simulink model "Md61StEnCtrl"  (R2018b)
settings: Solver=FixedStepDiscrete  StartTime=0.0  StopTime=10.0  RelTol=1e-3
undefined symbols (not defined in the file or in its folder): data, KeSMSuFirstRwStBackPosDelta_Val, KeSMSuThrdRwCushFoldPosDelta_Val, KeSMSwAcsMd30PassStFldUpwdDnwdPos1_Val, KeSMSwAcsMd30PassStFrwdBkwdPos1_Val, KeSMSwAcsMd31PassStBkReclnUpwdDnwdPos1_Val, KeSMSwSeatBkLimitPos_Val, KeSMSwSeatBkLimitPosDelt_Val, PassStBkReclnEn_Clear, PassStBkReclnEn_Set, PassStCshnFldEn_Clear, PassStCshnFldEn_Set, PassStFwdBkwdEn_Clear, PassStFwdBkwdEn_Set, SecRwLtStBkReclnEn_Clear, SecRwLtStBkReclnEn_Set, SecRwLtStFwdBkwdEn_Clear, SecRwLtStFwdBkwdEn_Set, SecRwLtStLgrstInwdOtwdEn_Clear, SecRwLtStLgrstInwdOtwdEn_Set, SecRwLtStLgrstUpwdDnwdEn_Clear, SecRwLtStLgrstUpwdDnwdEn_Set, SecRwRtStBkReclnEn_Clear, SecRwRtStBkReclnEn_Set, SecRwRtStFwdBkwdEn_Clear, SecRwRtStFwdBkwdEn_Set, SecRwRtStLgrstInwdOtwdEn_Clear, SecRwRtStLgrstInwdOtwdEn_Set, SecRwRtStLgrstUpwdDnwdEn_Clear, SecRwRtStLgrstUpwdDnwdEn_Set, ThdRwLtStBkReclnEn_Clear, ThdRwLtStBkReclnEn_Set, ThdRwLtStCshnFldEn_Clear, ThdRwLtStCshnFldEn_Set, ThdRwLtStFwdBkwdEn_Clear, ThdRwLtStFwdBkwdEn_Set, ThdRwRtStBkReclnEn_Clear, ThdRwRtStBkReclnEn_Set, ThdRwRtStCshnFldEn_Clear, ThdRwRtStCshnFldEn_Set, ThdRwRtStFwdBkwdEn_Clear, ThdRwRtStFwdBkwdEn_Set, ZeroLEn_Clear, ZeroLEn_Set, ZeroREn_Clear, ZeroREn_Set
libraries: simulink x1
(part 2 of 3)

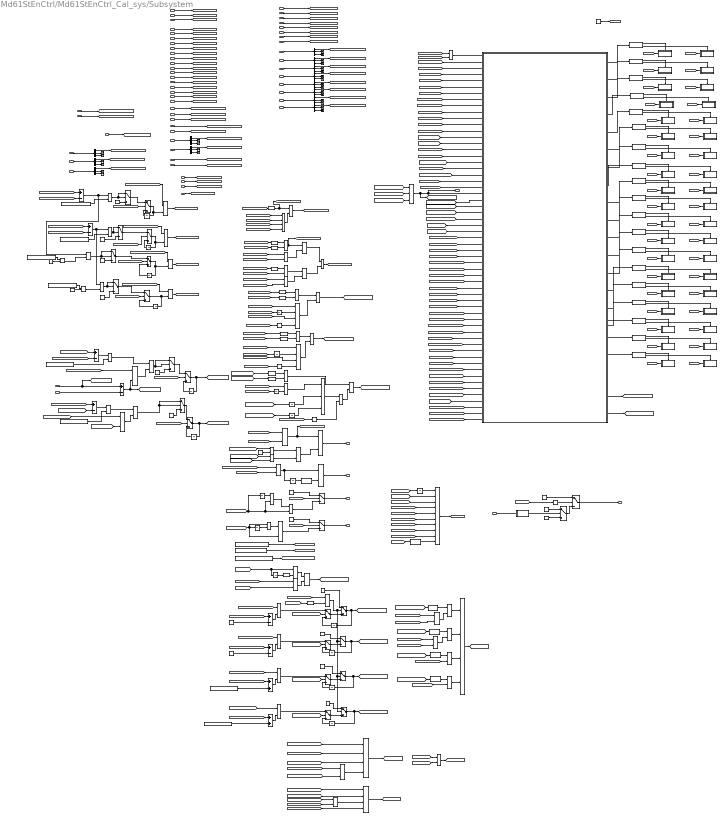
== system Md61StEnCtrl/Md61StEnCtrl_Cal_sys/Subsystem ==
  note: 3.13.1
  note: 3.13.1新增条件
  note: 3.13.1
  MdXXIsTargetPosZone_Val_read : Inport
  PassStBkReclnStgDone_Val_read : Inport  Port=2
  PassStCshnFldStgDone_Val_read : Inport  Port=3
  PassStFwdBkwdStgDone_Val_read : Inport  Port=4
  SecRwLtStBkReclnStgDone_Val_read : Inport  Port=5
  SecRwLtStFrwdBkwdStgDone_Val_read : Inport  Port=6
  SecRwLtStLgrstOtwdInwdStgDone_Val_read : Inport  Port=7
  SecRwLtStLgrstUpwdDnwdStgDone_Val_read : Inport  Port=8
  SecRwRtStBkReclnStgDone_Val_read : Inport  Port=9
  SecRwRtStFrwdBkwdStgDone_Val_read : Inport  Port=10
  SecRwRtStLgrstOtwdInwdStgDone_Val_read : Inport  Port=11
  SecRwRtStLgrstUpwdDnwdStgDone_Val_read : Inport  Port=12
  ThdRwLtStBkReclnStgDone_Val_read : Inport  Port=13
  ThdRwLtStCshnFldStgDone_Val_read : Inport  Port=14
  ThdRwLtStFwdBkwdStgDone_Val_read : Inport  Port=15
  ThdRwRtStBkReclnStgDone_Val_read : Inport  Port=16
  ThdRwRtStCshnFldStgDone_Val_read : Inport  Port=17
  ThdRwRtStFwdBkwdStgDone_Val_read : Inport  Port=18
  ZeroLStgDone_Val_read : Inport  Port=19
  ZeroRStgDone_Val_read : Inport  Port=20
  IfVeSMSbThdRwLtStCshnFldUpwdDnwdMovConfig_Val_read : Inport  Port=21
  IfVeSMSbThdRwRtStCshnFldUpwdDnwdMovConfig_Val_read : Inport  Port=22
  IfVeSMSuPassStFldUpwdDnwdPos_Val_read : Inport  Port=23
  IfVeSMSuPassStFrwdBkwdPos_Val_read : Inport  Port=24
  IfVeSMSuThdRwLtStCshnFldUpwdDnwdPos_Val_read : Inport  Port=25
  IfVeSMSuThdRwLtStFrwdBkwdPos_Val_read : Inport  Port=26
  IfVeSMSuThdRwRtStCshnFldUpwdDnwdPos_Val_read : Inport  Port=27
  IfVeSMSuThdRwRtStFrwdBkwdPos_Val_read : Inport  Port=28
  Md61ThdRwLtStCshnFldTrgtPosCalib_TrgtPosArray_read : Inport  Port=29
  Md61ThdRwRtStCshnFldTrgtPosCalib_TrgtPosArray_read : Inport  Port=30
  Md61PassStNeedFldOpn_Val_read : Inport  Port=31
  Md61ThdRwLtStNeedFldOpn_Val_read : Inport  Port=32
  Md61ThdRwRtStNeedFldOpn_Val_read : Inport  Port=33
  FirstTrig : Inport  Port=34
  KeSMSwSeatBkLimitPos_Val : Inport  Port=35
  KeSMSwSeatBkLimitPosDelt_Val : Inport  Port=36
  IfVeSMSuPassStBkReclnUpwdDnwdPos_Val_read : Inport  Port=37
  Md61PassStBkReclnTrgtPos_Val_read : Inport  Port=38
  Md61PassStFwdBkwdTrgtPosCalib_TrgtPosArray_read : Inport  Port=39
  Md61ThdRwLtStFrwdBkwdPosTrgtPosCalib_TrgtPosArray_read : Inport  Port=40
  Md61ThdRwRtStFrwdBkwdPosTrgtPosCalib_TrgtPosArray_read : Inport  Port=41
  IfVeSMSuSecRwLtStBkReclnUpwdDnwdPos_Val_read : Inport  Port=42
  IfVeSMSuSecRwLtStLgrstOtwdInwdPos_Val_read : Inport  Port=43
  IfVeSMSuSecRwLtStLgrstUpwdDnwdPos_Val_read : Inport  Port=44
  IfVeSMSuSecRwLtStZeroPos_Val_read : Inport  Port=45
  IfVeSMSuSecRwRtStBkReclnUpwdDnwdPos_Val_read : Inport  Port=46
  IfVeSMSuSecRwRtStLgrstOtwdInwdPos_Val_read : Inport  Port=47
  IfVeSMSuSecRwRtStLgrstUpwdDnwdPos_Val_read : Inport  Port=48
  IfVeSMSuSecRwRtStZeroPos_Val_read : Inport  Port=49
  Md61SecRwLtStBkReclnTrgtPosCalib_TrgtPosArray_read : Inport  Port=50
  Md61SecRwLtStCushFrntTrgtPosCalib_TrgtPosArray_read : Inport  Port=51
  Md61SecRwLtStLgrstInwdOtwdTrgtPosCalib_TrgtPosArray_read : Inport  Port=52
  Md61SecRwLtStLgrstUpwdDnwdTrgtPosCalib_TrgtPosArray_read : Inport  Port=53
  Md61SecRwRtStBkReclnTrgtPosCalib_TrgtPosArray_read : Inport  Port=54
  Md61SecRwRtStCushFrntTrgtPosCalib_TrgtPosArray_read : Inport  Port=55
  Md61SecRwRtStLgrstInwdOtwdTrgtPosCalib_TrgtPosArray_read : Inport  Port=56
  Md61SecRwRtStLgrstUpwdDnwdTrgtPosCalib_TrgtPosArray_read : Inport  Port=57
  32BitSelector1 : Subsystem  mask(32 Bit Selector){BitNum=5}
      mask prompts: BitNum "Select Bit Number"
      mask help: Allows selection of a particular bit (0-31) out of a packed word up to 32 bits long. Output will be true if the bit number selected via the mask parameter is equal to one.
      mask TypeOptions BitNum: 0 | 1 | 2 | 3 | 4 | 5 | 6 | 7 | 8 | 9 | 10 | 11 | 12 | 13 | 14 | 15 | 16 | 17 | 18 | 19 | 20 | 21 | 22 | 23 | 24 | 25 | 26 | 27 | 28 | 29 | 30 | 31
      mask Display:
      | text(0.5, 0.8,'BIT','horizontalAlignment','center')
      | text(0.5, 0.5,'SELECTOR','horizontalAlignment','center')
      | text(0.5, 0.2,['-- Bit ',char(get_param(gcb,'BitNum')),' --'],'horizontalAlignment','center')
  Add{,1,3..5,7} (6 alike) : Sum  Inputs=+-  AccumDataTypeStr=int16  OutDataTypeStr=int16
  Add2 : Sum  Inputs=+-  OutDataTypeStr=int16
  Add6 : Sum  OutDataTypeStr=int16
  Add8 : Sum  OutDataTypeStr=int16
  Chart : Stateflow chart  TreatAsAtomicUnit=on
  Constant : Constant  OutDataTypeStr=uint8
  Constant1 : Constant  Value=2  OutDataTypeStr=uint8
  Constant{10..11,16..20,22..26} (12 alike) : Constant  Value=0  OutDataTypeStr=boolean
  Constant12 : Constant  Value=120  OutDataTypeStr=int16
  Constant13 : Constant  Value=120  OutDataTypeStr=int16
  Constant2 : Constant  Value=0  OutDataTypeStr=uint8
  Constant3 : Constant  Value=5  OutDataTypeStr=uint8
  Constant4 : Constant  Value=-1  OutDataTypeStr=int16
  Constant5 : Constant  Value=-1  OutDataTypeStr=int16
  Constant9 : Constant  Value=120  OutDataTypeStr=uint16
  Demux{,1..12} (13 alike) : Demux  Outputs=3
  Divide : Product  Inputs=**  OutDataTypeStr=int16
  Divide1 : Product  Inputs=**  OutDataTypeStr=int16
  If{1..19} (19 alike) : If  IfExpression=u1
  Logical Operator{,6,11,21,26,41,51..54,68,74} (12 alike) : Logic  Operator=OR  AllPortsSameDT=off  OutDataTypeStr=boolean
  Logical Operator{1,3..4,7,10,22..23,27..28,34..35,42,46..47,49..50,55..57,70..72} (22 alike) : Logic  Operator=NOT  AllPortsSameDT=off  OutDataTypeStr=boolean
  Logical Operator{5,8..9,12..19,24,31..33,37,39..40,43..45,48,58..59,62,64..65,67,69,73} (30 alike) : Logic  AllPortsSameDT=off  OutDataTypeStr=boolean
  Logical Operator{2,20,25,60..61,63} (6 alike) : Logic  Inputs=4  AllPortsSameDT=off  OutDataTypeStr=boolean
  Logical Operator36 : Logic  Operator=OR  Inputs=3  AllPortsSameDT=off  OutDataTypeStr=boolean
  Logical Operator38 : Logic  Inputs=3  AllPortsSameDT=off  OutDataTypeStr=boolean
  Logical Operator66 : Logic  Inputs=10  AllPortsSameDT=off  OutDataTypeStr=boolean
  PA_KeSMSuFirstRwStBackPosDelta_Val{,1..3} (4 alike) : Constant  Value=KeSMSuFirstRwStBackPosDelta_Val
  PA_KeSMSuThrdRwCushFoldPosDelta_Val{,1..3} (4 alike) : Constant  Value=KeSMSuThrdRwCushFoldPosDelta_Val
  PA_KeSMSwAcsMd30PassStFldUpwdDnwdPos1_Val : Constant  Value=KeSMSwAcsMd30PassStFldUpwdDnwdPos1_Val
  PA_KeSMSwAcsMd30PassStFrwdBkwdPos1_Val : Constant  Value=KeSMSwAcsMd30PassStFrwdBkwdPos1_Val
  PA_KeSMSwAcsMd31PassStBkReclnUpwdDnwdPos1_Val : Constant  Value=KeSMSwAcsMd31PassStBkReclnUpwdDnwdPos1_Val
  PassStBkRecln_Clear : Subsystem  TreatAsAtomicUnit=on
  PassStBkRecln_Set : Subsystem  TreatAsAtomicUnit=on
  PassStCshnFld_Clear : Subsystem  TreatAsAtomicUnit=on
  PassStCshnFld_Set : Subsystem  TreatAsAtomicUnit=on
  PassStFwdBkwd_Clear : Subsystem  TreatAsAtomicUnit=on
  PassStFwdBkwd_Set : Subsystem  TreatAsAtomicUnit=on
  Relational Operator{,1,4,14..16} (6 alike) : RelationalOperator  Operator=>  OutDataTypeStr=boolean  RndMeth=Simplest
  Relational Operator10 : RelationalOperator  Operator=~=  OutDataTypeStr=boolean  RndMeth=Simplest
  Relational Operator11 : RelationalOperator  Operator=~=  OutDataTypeStr=boolean  RndMeth=Simplest
  Relational Operator{2..3,5..6,12..13} (6 alike) : RelationalOperator  Operator=<  OutDataTypeStr=boolean  RndMeth=Simplest
  Relational Operator7 : RelationalOperator  Operator=<=  OutDataTypeStr=boolean  RndMeth=Simplest
  Relational Operator8 : RelationalOperator  OutDataTypeStr=boolean  RndMeth=Simplest
  Relational Operator9 : RelationalOperator  Operator=<=  OutDataTypeStr=boolean  RndMeth=Simplest
  SecRwLtStBkRecln_Clear : Subsystem  TreatAsAtomicUnit=on
  SecRwLtStBkRecln_Set : Subsystem  TreatAsAtomicUnit=on
  SecRwLtStFwdBkwd_Clear : Subsystem  TreatAsAtomicUnit=on
  SecRwLtStFwdBkwd_Set : Subsystem  TreatAsAtomicUnit=on
  SecRwLtStLgrstInwdOtwd_Clear : Subsystem  TreatAsAtomicUnit=on
  SecRwLtStLgrstInwdOtwd_Set : Subsystem  TreatAsAtomicUnit=on
  SecRwLtStLgrstUpwdDnwd_Clear : Subsystem  TreatAsAtomicUnit=on
  SecRwLtStLgrstUpwdDnwd_Set : Subsystem  TreatAsAtomicUnit=on
  SecRwRtStBkRecln_Clear : Subsystem  TreatAsAtomicUnit=on
  SecRwRtStBkRecln_Set : Subsystem  TreatAsAtomicUnit=on
  SecRwRtStFwdBkwd_Clear : Subsystem  TreatAsAtomicUnit=on
  SecRwRtStFwdBkwd_Set : Subsystem  TreatAsAtomicUnit=on
  SecRwRtStLgrstInwdOtwd_Clear : Subsystem  TreatAsAtomicUnit=on
  SecRwRtStLgrstInwdOtwd_Set : Subsystem  TreatAsAtomicUnit=on
  SecRwRtStLgrstUpwdDnwd_Clear : Subsystem  TreatAsAtomicUnit=on
  SecRwRtStLgrstUpwdDnwd_Set : Subsystem  TreatAsAtomicUnit=on
  Switch{,1..5,8..13,18..21} (16 alike) : Switch  Criteria=u2 > Threshold
  Switch{6..7,14..17,22..23} (8 alike) : Switch  Criteria=u2 > Threshold  OutDataTypeStr=boolean
  Terminator{,1..25} (26 alike) : Terminator
  ThdRwLtStBkRecln_Clear : Subsystem  TreatAsAtomicUnit=on
  ThdRwLtStBkRecln_Set : Subsystem  TreatAsAtomicUnit=on
  ThdRwLtStCshnFld_Clear : Subsystem  TreatAsAtomicUnit=on
  ThdRwLtStCshnFld_Set : Subsystem  TreatAsAtomicUnit=on
  ThdRwLtStFwdBkwd_Clear : Subsystem  TreatAsAtomicUnit=on
  ThdRwLtStFwdBkwd_Set : Subsystem  TreatAsAtomicUnit=on
  ThdRwRtStBkRecln_Clear : Subsystem  TreatAsAtomicUnit=on
  ThdRwRtStBkRecln_Set : Subsystem  TreatAsAtomicUnit=on
  ThdRwRtStCshnFld_Clear : Subsystem  TreatAsAtomicUnit=on
  ThdRwRtStCshnFld_Set : Subsystem  TreatAsAtomicUnit=on
  ThdRwRtStFwdBkwd_Clear : Subsystem  TreatAsAtomicUnit=on
  ThdRwRtStFwdBkwd_Set : Subsystem  TreatAsAtomicUnit=on
  Unit Delay{,1..19} (20 alike) : UnitDelay  SampleTime=-1
  ZeroL_Clear : Subsystem  TreatAsAtomicUnit=on
  ZeroL_Set : Subsystem  TreatAsAtomicUnit=on
  ZeroR_Clear : Subsystem  TreatAsAtomicUnit=on
  ZeroR_Set : Subsystem  TreatAsAtomicUnit=on
  Md61MdDone_Val_write : Outport
      settings: EnsureOutportIsVirtual=on
  Md61PassBkReset_Val_write : Outport  Port=2
      settings: EnsureOutportIsVirtual=on
  Md61PassFwdBkwdReset_Val_write : Outport  Port=3
      settings: EnsureOutportIsVirtual=on
  Md61Stage2DoneSecRwStReset_Val_write : Outport  Port=4
      settings: EnsureOutportIsVirtual=on
  Md61ThdRwLtStFwdBkwdReset_Val_write : Outport  Port=5
      settings: EnsureOutportIsVirtual=on
  Md61ThdRwRtStFwdBkwdReset_Val_write : Outport  Port=6
      settings: EnsureOutportIsVirtual=on
  wires:
  Switch/1 -> Md61MdDone_Val_write/1
  Constant/1 -> Switch1/1
  Constant1/1 -> Switch1/3
  [AllDone] -> Logical Operator7/1
  MdXXIsTargetPosZone_Val_read/1 -> 32BitSelector1/1(x)
  32BitSelector1/1(y) -> Switch1/2
  Constant2/1 -> Switch/1
  Logical Operator7/1 -> Switch/2
  Switch1/1 -> Switch/3
  If6/1 -> PassStBkRecln_Set/Action
  If6/2 -> PassStBkRecln_Clear/Action
  Constant3/1 -> [Mdbit]
  [Mdbit] -> PassStBkRecln_Set/1(MdBitNum)
  [Mdbit] -> PassStBkRecln_Clear/1(MdBitNum)
  [Mdbit] -> PassStCshnFld_Clear/1(MdBitNum)
  [Mdbit] -> PassStCshnFld_Set/1(MdBitNum)
  If1/2 -> PassStCshnFld_Clear/Action
  If1/1 -> PassStCshnFld_Set/Action
  If2/1 -> PassStFwdBkwd_Set/Action
  [Mdbit] -> PassStFwdBkwd_Set/1(MdBitNum)
  If2/2 -> PassStFwdBkwd_Clear/Action
  [Mdbit] -> PassStFwdBkwd_Clear/1(MdBitNum)
  [Mdbit] -> SecRwLtStBkRecln_Clear/1(MdBitNum)
  If3/2 -> SecRwLtStBkRecln_Clear/Action
  [Mdbit] -> SecRwLtStBkRecln_Set/1(MdBitNum)
  If3/1 -> SecRwLtStBkRecln_Set/Action
  [Mdbit] -> SecRwLtStFwdBkwd_Clear/1(MdBitNum)
  If4/2 -> SecRwLtStFwdBkwd_Clear/Action
  [Mdbit] -> SecRwLtStFwdBkwd_Set/1(MdBitNum)
  If4/1 -> SecRwLtStFwdBkwd_Set/Action
  [Mdbit] -> SecRwLtStLgrstInwdOtwd_Clear/1(MdBitNum)
  If5/2 -> SecRwLtStLgrstInwdOtwd_Clear/Action
  [Mdbit] -> SecRwLtStLgrstInwdOtwd_Set/1(MdBitNum)
  If5/1 -> SecRwLtStLgrstInwdOtwd_Set/Action
  [Mdbit] -> SecRwLtStLgrstUpwdDnwd_Clear/1(MdBitNum)
  If7/2 -> SecRwLtStLgrstUpwdDnwd_Clear/Action
  [Mdbit] -> SecRwLtStLgrstUpwdDnwd_Set/1(MdBitNum)
  If7/1 -> SecRwLtStLgrstUpwdDnwd_Set/Action
  [Mdbit] -> SecRwRtStBkRecln_Clear/1(MdBitNum)
  If8/2 -> SecRwRtStBkRecln_Clear/Action
  [Mdbit] -> SecRwRtStBkRecln_Set/1(MdBitNum)
  If8/1 -> SecRwRtStBkRecln_Set/Action
  [Mdbit] -> SecRwRtStFwdBkwd_Clear/1(MdBitNum)
  If9/2 -> SecRwRtStFwdBkwd_Clear/Action
  [Mdbit] -> SecRwRtStFwdBkwd_Set/1(MdBitNum)
  If9/1 -> SecRwRtStFwdBkwd_Set/Action
  [Mdbit] -> SecRwRtStLgrstInwdOtwd_Clear/1(MdBitNum)
  If10/2 -> SecRwRtStLgrstInwdOtwd_Clear/Action
  [Mdbit] -> SecRwRtStLgrstInwdOtwd_Set/1(MdBitNum)
  If10/1 -> SecRwRtStLgrstInwdOtwd_Set/Action
  [Mdbit] -> SecRwRtStLgrstUpwdDnwd_Clear/1(MdBitNum)
  If11/2 -> SecRwRtStLgrstUpwdDnwd_Clear/Action
  [Mdbit] -> SecRwRtStLgrstUpwdDnwd_Set/1(MdBitNum)
  If11/1 -> SecRwRtStLgrstUpwdDnwd_Set/Action
  [Mdbit] -> ThdRwLtStBkRecln_Clear/1(MdBitNum)
  If12/2 -> ThdRwLtStBkRecln_Clear/Action
  [Mdbit] -> ThdRwLtStBkRecln_Set/1(MdBitNum)
  If12/1 -> ThdRwLtStBkRecln_Set/Action
  [Mdbit] -> ThdRwLtStCshnFld_Clear/1(MdBitNum)
  If13/2 -> ThdRwLtStCshnFld_Clear/Action
  [Mdbit] -> ThdRwLtStCshnFld_Set/1(MdBitNum)
  If13/1 -> ThdRwLtStCshnFld_Set/Action
  [Mdbit] -> ThdRwLtStFwdBkwd_Clear/1(MdBitNum)
  If14/2 -> ThdRwLtStFwdBkwd_Clear/Action
  [Mdbit] -> ThdRwLtStFwdBkwd_Set/1(MdBitNum)
  If14/1 -> ThdRwLtStFwdBkwd_Set/Action
  [Mdbit] -> ThdRwRtStBkRecln_Clear/1(MdBitNum)
  If15/2 -> ThdRwRtStBkRecln_Clear/Action
  [Mdbit] -> ThdRwRtStBkRecln_Set/1(MdBitNum)
  If15/1 -> ThdRwRtStBkRecln_Set/Action
  [Mdbit] -> ThdRwRtStCshnFld_Clear/1(MdBitNum)
  If16/2 -> ThdRwRtStCshnFld_Clear/Action
  [Mdbit] -> ThdRwRtStCshnFld_Set/1(MdBitNum)
  If16/1 -> ThdRwRtStCshnFld_Set/Action
  [Mdbit] -> ThdRwRtStFwdBkwd_Clear/1(MdBitNum)
  If17/2 -> ThdRwRtStFwdBkwd_Clear/Action
  [Mdbit] -> ThdRwRtStFwdBkwd_Set/1(MdBitNum)
  If17/1 -> ThdRwRtStFwdBkwd_Set/Action
  [Mdbit] -> ZeroL_Clear/1(MdBitNum)
  If18/2 -> ZeroL_Clear/Action
  [Mdbit] -> ZeroL_Set/1(MdBitNum)
  If18/1 -> ZeroL_Set/Action
  [Mdbit] -> ZeroR_Clear/1(MdBitNum)
  If19/2 -> ZeroR_Clear/Action
  [Mdbit] -> ZeroR_Set/1(MdBitNum)
  If19/1 -> ZeroR_Set/Action
  Chart/1(PassStBkReclnEn) -> If6/1
  Chart/2(PassStCshnFldEn) -> If1/1
  Chart/3(PassStFwdBkwdEn) -> If2/1
  Chart/4(SecRwLtStBkReclnEn) -> If3/1
  Chart/5(SecRwLtStFwdBkwdEn) -> If4/1
  Chart/6(SecRwLtStLgrstInwdOtwdEn) -> If5/1
  Chart/7(SecRwLtStLgrstUpwdDnwdEn) -> If7/1
  Chart/8(SecRwRtStBkReclnEn) -> If8/1
  Chart/9(SecRwRtStFwdBkwdEn) -> If9/1
  Chart/10(SecRwRtStLgrstInwdOtwdEn) -> If10/1
  Chart/11(SecRwRtStLgrstUpwdDnwdEn) -> If11/1
  Chart/12(ThdRwLtStBkReclnEn) -> If12/1
  Chart/13(ThdRwLtStCshnFldEn) -> If13/1
  Chart/14(ThdRwLtStFwdBkwdEn) -> If14/1
  Chart/15(ThdRwRtStBkReclnEn) -> If15/1
  Chart/16(ThdRwRtStCshnFldEn) -> If16/1
  Chart/17(ThdRwRtStFwdBkwdEn) -> If17/1
  Chart/18(ZeroLEn) -> If18/1
  Chart/19(ZeroREn) -> If19/1
  IfVeSMSbThdRwLtStCshnFldUpwdDnwdMovConfig_Val_read/1 -> [ThdRwLtStCshnFldUpwdDnwdMovConfig]
  IfVeSMSbThdRwRtStCshnFldUpwdDnwdMovConfig_Val_read/1 -> [ThdRwRtStCshnFldUpwdDnwdMovConfig]
  IfVeSMSuPassStFldUpwdDnwdPos_Val_read/1 -> [IfVeSMSuPassStFldUpwdDnwdPos]
  IfVeSMSuPassStFrwdBkwdPos_Val_read/1 -> [IfVeSMSuPassStFrwdBkwdPos]
  IfVeSMSuThdRwLtStCshnFldUpwdDnwdPos_Val_read/1 -> [IfVeSMSuThdRwLtStCshnFldUpwdDnwdPos]
  IfVeSMSuThdRwRtStCshnFldUpwdDnwdPos_Val_read/1 -> [IfVeSMSuThdRwRtStCshnFldUpwdDnwdPos]
  IfVeSMSuThdRwRtStFrwdBkwdPos_Val_read/1 -> [ThdRwRtStFrwdBkwdPos]
  Md61ThdRwLtStCshnFldTrgtPosCalib_TrgtPosArray_read/1 -> Demux/1
  Md61ThdRwRtStCshnFldTrgtPosCalib_TrgtPosArray_read/1 -> Demux2/1
  Logical Operator1/1 -> [Md61ThdRwLtStNotNeedFldOpn], Logical Operator/1
  SecRwLtStBkReclnStgDone_Val_read/1 -> [SecRwLtStBkReclnStgDone]
  SecRwLtStFrwdBkwdStgDone_Val_read/1 -> [SecRwLtStFrwdBkwdStgDone]
  SecRwLtStLgrstOtwdInwdStgDone_Val_read/1 -> [SecRwLtStLgrstOtwdInwdStgDone]
  SecRwLtStLgrstUpwdDnwdStgDone_Val_read/1 -> [SecRwLtStLgrstUpwdDnwdStgDone]
  PassStBkReclnStgDone_Val_read/1 -> [PassStBkReclnStgDone]
  PassStCshnFldStgDone_Val_read/1 -> [PassStCshnFldStgDone]
  PassStFwdBkwdStgDone_Val_read/1 -> [PassStFwdBkwdStgDone]
  SecRwRtStBkReclnStgDone_Val_read/1 -> [SecRwRtStBkReclnStgDone]
  SecRwRtStFrwdBkwdStgDone_Val_read/1 -> [SecRwRtStFrwdBkwdStgDone]
  SecRwRtStLgrstOtwdInwdStgDone_Val_read/1 -> [SecRwRtStLgrstOtwdInwdStgDone]
  SecRwRtStLgrstUpwdDnwdStgDone_Val_read/1 -> [SecRwRtStLgrstUpwdDnwdStgDone]
  ThdRwLtStBkReclnStgDone_Val_read/1 -> [ThdRwLtStBkReclnStgDone]
  ThdRwLtStCshnFldStgDone_Val_read/1 -> [ThdRwLtStCshnFldStgDone]
  ThdRwLtStFwdBkwdStgDone_Val_read/1 -> [ThdRwLtStFwdBkwdStgDone]
  ThdRwRtStBkReclnStgDone_Val_read/1 -> [ThdRwRtStBkReclnStgDone]
  ThdRwRtStCshnFldStgDone_Val_read/1 -> [ThdRwRtStCshnFldStgDone]
  ThdRwRtStFwdBkwdStgDone_Val_read/1 -> [ThdRwRtStFwdBkwdStgDone]
  ZeroLStgDone_Val_read/1 -> [ZeroLStgDone]
  ZeroRStgDone_Val_read/1 -> [ZeroRStgDone]
  Logical Operator2/1 -> Logical Operator/2
  [SecRwLtStBkReclnStgDone] -> Logical Operator2/1
  [SecRwLtStFrwdBkwdStgDone] -> Logical Operator2/2
  [SecRwLtStLgrstOtwdInwdStgDone] -> Logical Operator2/3
  [SecRwLtStLgrstUpwdDnwdStgDone] -> Logical Operator2/4
  Logical Operator/1 -> [Stage1SecRwLtStDone]
  Md61ThdRwLtStNeedFldOpn_Val_read/1 -> [Md61ThdRwLtStNeedFldOpn]
  [Md61ThdRwLtStNeedFldOpn] -> Logical Operator1/1
  Md61ThdRwRtStNeedFldOpn_Val_read/1 -> [Md61ThdRwRtStNeedFldOpn]
  Md61PassStNeedFldOpn_Val_read/1 -> [Md61PassStNeedFldOpn]
  [Md61ThdRwLtStNeedFldOpn] -> Logical Operator3/1
  [Md61ThdRwRtStNeedFldOpn] -> Logical Operator4/1
  Logical Operator3/1 -> Logical Operator5/1
  Logical Operator4/1 -> Logical Operator5/2
  Logical Operator5/1 -> [Md61ThdRwNotNeedFldOpn], Logical Operator6/1
  [SecRwRtStFrwdBkwdStgDone] -> Logical Operator8/2
  [SecRwRtStBkReclnStgDone] -> Logical Operator8/1
  Logical Operator8/1 -> Logical Operator6/2
  FirstTrig/1 -> [FirstTrig]
  Logical Operator10/1 -> Logical Operator9/1
  [Md61PassStNeedFldOpn] -> Logical Operator10/1
  [Md61ThdRwNotNeedFldOpn] -> Logical Operator9/2
  Logical Operator9/1 -> Logical Operator11/1
  [SecRwRtStLgrstUpwdDnwdStgDone] -> Logical Operator12/2
  [SecRwRtStLgrstOtwdInwdStgDone] -> Logical Operator12/1
  Logical Operator12/1 -> Logical Operator11/2
  Logical Operator6/1 -> Logical Operator13/1
  Logical Operator11/1 -> Logical Operator13/2
  Logical Operator13/1 -> [Stage1SecRwRtStDone]
  [Stage1SecRwLtStDone] -> Logical Operator14/1
  [Stage1SecRwRtStDone] -> Logical Operator14/2
  [Md61ThdRwNotNeedFldOpn] -> Chart/2(Md61ThdRwNotNeedFldOpn)
  Logical Operator14/1 -> Chart/1(Stage1SecRwDone)
  Demux/1 -> [Md61ThdRwLtStCshnFldTrgtPos]
  Demux/2 -> Terminator/1
  Demux/3 -> Terminator1/1
  Demux2/3 -> Terminator5/1
  Demux2/2 -> Terminator4/1
  Demux2/1 -> [Md61ThdRwRtStCshnFldTrgtPos]
  [Md61ThdRwLtStNotNeedFldOpn] -> Chart/3(Md61ThdRwLtStNotNeedFldOpn)
  Switch2/1 -> Unit Delay/1, Logical Operator15/2
  Unit Delay/1 -> Switch2/3
  Logical Operator15/1 -> [ThdRwLtNeedFld]
  [FirstTrig] -> Switch5/2
  [FirstTrig] -> Switch2/2
  [FirstTrig] -> Switch4/2
  Logical Operator17/1 -> [ThdRwRtNeedFld]
  Unit Delay1/1 -> Switch3/3
  [IfVeSMSuThdRwLtStCshnFldUpwdDnwdPos] -> Add/1
  Add1/1 -> Relational Operator3/1, Relational Operator1/1
  [ThdRwRtStCshnFldUpwdDnwdMovConfig] -> Logical Operator17/1
  PA_KeSMSuThrdRwCushFoldPosDelta_Val1/1 -> Relational Operator1/2
  Add/1 -> Relational Operator/1, Relational Operator2/1
  Divide1/1 -> Relational Operator3/2
  [IfVeSMSuThdRwRtStCshnFldUpwdDnwdPos] -> Add1/1
  Logical Operator16/1 -> [ThdRwLtNeedOpn]
  Switch5/1 -> Unit Delay3/1, Logical Operator18/2
  [ThdRwLtStCshnFldUpwdDnwdMovConfig] -> Logical Operator16/1
  Unit Delay3/1 -> Switch5/3
  [FirstTrig] -> Switch3/2
  Switch3/1 -> Logical Operator17/2, Unit Delay1/1
  Switch4/1 -> Logical Operator16/2, Unit Delay2/1
  [ThdRwRtStCshnFldUpwdDnwdMovConfig] -> Logical Operator18/1
  [Md61ThdRwRtStCshnFldTrgtPos] -> Add1/2
  [Md61ThdRwLtStCshnFldTrgtPos] -> Add/2
  Unit Delay2/1 -> Switch4/3
  [ThdRwLtStCshnFldUpwdDnwdMovConfig] -> Logical Operator15/1
  Logical Operator18/1 -> [ThdRwRtNeedOpn]
  Relational Operator1/1 -> Switch18/1, Switch18/2
  [ThdRwLtStBkReclnStgDone] -> Logical Operator20/1
  [ThdRwLtStCshnFldStgDone] -> Unit Delay11/1
  Logical Operator24/1 -> Logical Operator26/1
  [ThdRwRtNeedOpn] -> Logical Operator27/1
  Logical Operator27/1 -> Logical Operator24/1
  [ThdRwRtNeedFld] -> Logical Operator28/1
  Logical Operator28/1 -> Logical Operator24/2
  [ThdRwRtStBkReclnStgDone] -> Logical Operator25/1
  [ThdRwRtStCshnFldStgDone] -> Unit Delay10/1
  [ThdRwRtStFwdBkwdStgDone] -> Logical Operator25/3
  Logical Operator25/1 -> Logical Operator26/2
  Logical Operator26/1 -> [Stage2ThdRwRtDone]
  Logical Operator23/1 -> Logical Operator19/2
  [ThdRwLtNeedFld] -> Logical Operator23/1
  Logical Operator22/1 -> Logical Operator19/1
  [ThdRwLtNeedOpn] -> Logical Operator22/1
  Logical Operator19/1 -> Logical Operator21/1
  [ThdRwLtStFwdBkwdStgDone] -> Logical Operator20/3
  Logical Operator20/1 -> Logical Operator21/2
  Logical Operator21/1 -> [Stage2ThdRwLtDone]  "Stage2ThdRwLtDone"
  [ThdRwLtNeedOpn] -> Chart/6(ThdRwLtNeedOpn)
  [ThdRwRtNeedOpn] -> Chart/7(ThdRwRtNeedOpn)
  [ThdRwLtNeedFld] -> Chart/4(ThdRwLtNeedFld)
  [ThdRwRtNeedFld] -> Chart/5(ThdRwRtNeedFld)
  [ThdRwLtStCshnFldStgDone] -> Chart/8(ThdRwLtStCshnFldStgDone)
  [ThdRwLtStBkReclnStgDone] -> Chart/9(ThdRwLtStBkReclnStgDone)
  [ThdRwRtStCshnFldStgDone] -> Chart/10(ThdRwRtStCshnFldStgDone)
  [ThdRwRtStBkReclnStgDone] -> Chart/11(ThdRwRtStBkReclnStgDone)
  [ThdRwLtStFwdBkwdStgDone] -> Chart/12(ThdRwLtStFwdBkwdStgDone)
  [ThdRwRtStFwdBkwdStgDone] -> Chart/13(ThdRwRtStFwdBkwdStgDone)
  PA_KeSMSuFirstRwStBackPosDelta_Val/1 -> Relational Operator16/2
  Relational Operator16/1 -> Logical Operator31/1
  [Md61PassStBkReclnUpwdDnwdTrgtPos] -> Add7/2
  Relational Operator6/1 -> Logical Operator31/2
  [Md61PassStBkReclnUpwdDnwdTrgtPos] -> Relational Operator6/1
  [PassStBkReclnPos] -> Add7/1
  Add7/1 -> Relational Operator16/1
  KeSMSwSeatBkLimitPos_Val/1 -> [SeatBkLimitPos], Add2/1
  KeSMSwSeatBkLimitPosDelt_Val/1 -> Add2/2
  Md61PassStBkReclnTrgtPos_Val_read/1 -> [Md61PassStBkReclnUpwdDnwdTrgtPos]
  IfVeSMSuPassStBkReclnUpwdDnwdPos_Val_read/1 -> [PassStBkReclnPos]
  Add3/1 -> Relational Operator4/1
  PA_KeSMSuFirstRwStBackPosDelta_Val1/1 -> Relational Operator4/2
  [Md61PassStBkReclnUpwdDnwdTrgtPos] -> Add3/1
  [PassStBkReclnPos] -> Add3/2
  [PassStBkReclnPos] -> Relational Operator5/1
  Relational Operator5/1 -> Logical Operator32/2
  [FirstTrig] -> Switch6/2
  Switch6/1 -> Unit Delay4/1, [PassStNeedFld]
  Unit Delay4/1 -> Switch6/3
  Unit Delay5/1 -> Switch7/3
  Switch7/1 -> [PassStNeedOpn], Unit Delay5/1
  [FirstTrig] -> Switch7/2
  [PassStNeedOpn] -> Chart/15(PassStNeedOpn)
  [PassStNeedFld] -> Chart/14(PassStNeedFld)
  [PassStFwdBkwdStgDone] -> Chart/16(PassStFwdBkwdStgDone)
  [PassStBkReclnStgDone] -> Chart/17(PassStBkReclnStgDone)
  [PassStCshnFldStgDone] -> Chart/19(PassStCshnFldStgDone)
  [PassStBkReclnPos] -> Chart/18(PassStBkReclnUpwdDnwdPos)
  Logical Operator35/1 -> Logical Operator33/2
  [PassStNeedOpn] -> Logical Operator35/1
  Logical Operator34/1 -> Logical Operator33/1
  [PassStNeedFld] -> Logical Operator34/1
  [PassStFwdBkwdStgDone] -> Logical Operator37/1
  Chart/21(PassStCshnFldFailflg) -> [PassStCshnFldFailflg]
  Chart/20(PassStFwdBkwdFailflg) -> [PassStFwdBkwdFailflg]
  [PassStCshnFldFailflg] -> Unit Delay17/1
  [PassStFwdBkwdFailflg] -> Unit Delay18/1
  [Stage2ThdRwRtDone] -> Logical Operator38/2
  [Stage2PassStDone] -> Logical Operator38/3
  [Stage2ThdRwLtDone] -> Logical Operator38/1
  Logical Operator39/1 -> [PassStBkStgDone], Logical Operator40/1
  [PassStBkReclnStgDone] -> Logical Operator39/1
  [PassStBkReclnPos] -> Relational Operator7/1
  Constant9/1 -> Relational Operator7/2
  [PassStCshnFldStgDone] -> Logical Operator39/2
  Relational Operator7/1 -> Logical Operator41/1
  Logical Operator41/1 -> Logical Operator40/2
  [PassStBkReclnPos] -> Relational Operator8/1
  [SeatBkLimitPosMinusDelt] -> Relational Operator8/2
  Relational Operator8/1 -> Logical Operator41/2
  [PassStBkStgDone] -> Unit Delay6/1
  Unit Delay6/1 -> Logical Operator37/2
  Logical Operator42/1 -> Logical Operator43/2
  Relational Operator9/1 -> Logical Operator43/1, Unit Delay7/1
  [IfVeSMSuPassStFldUpwdDnwdPos] -> Relational Operator9/1
  Unit Delay7/1 -> Logical Operator42/1
  [PassStCshnFldTrgtPos1] -> Relational Operator9/2
  Logical Operator43/1 -> Md61PassBkReset_Val_write/1
  Constant10/1 -> Switch8/1
  Logical Operator44/1 -> Switch8/3
  [ThdRwLtStCshnFldStgDone] -> Unit Delay8/1, Relational Operator10/2, Logical Operator44/2
  Unit Delay8/1 -> Relational Operator10/1
  Relational Operator10/1 -> Logical Operator44/1
  [FirstTrig] -> Switch8/2
  Switch8/1 -> Md61ThdRwLtStFwdBkwdReset_Val_write/1
  Relational Operator11/1 -> Logical Operator45/1
  [ThdRwRtStCshnFldStgDone] -> Relational Operator11/1, Logical Operator45/2, Unit Delay9/1
  Unit Delay9/1 -> Relational Operator11/2
  Switch9/1 -> Md61ThdRwRtStFwdBkwdReset_Val_write/1
  [FirstTrig] -> Switch9/2
  Logical Operator45/1 -> Switch9/3
  Constant11/1 -> Switch9/1
  Unit Delay10/1 -> Logical Operator25/2
  Unit Delay11/1 -> Logical Operator20/2
  Logical Operator46/1 -> Logical Operator25/4
  [FirstTrig] -> Logical Operator46/1
  Logical Operator47/1 -> Logical Operator20/4
  [FirstTrig] -> Logical Operator47/1
  [Md31PassStBkReclnUpwdDnwdPos1] -> Chart/20(Md31PassStBkReclnTrgtPos1)
  [PassStCshnFldTrgtPos1] -> Chart/21(PassStCshnFldTrgtPos1)
  [PassStPassStFrwdBkwdTrgtPos1] -> Chart/22(PassStFwdBkwdTrgtPos1)
  Logical Operator40/1 -> Md61PassFwdBkwdReset_Val_write/1
  PA_KeSMSwAcsMd30PassStFldUpwdDnwdPos1_Val/1 -> [PassStCshnFldTrgtPos1]
  PA_KeSMSwAcsMd30PassStFrwdBkwdPos1_Val/1 -> [PassStPassStFrwdBkwdTrgtPos1]
  PA_KeSMSwAcsMd31PassStBkReclnUpwdDnwdPos1_Val/1 -> [Md31PassStBkReclnUpwdDnwdPos1]
  IfVeSMSuThdRwLtStFrwdBkwdPos_Val_read/1 -> [ThdRwLtStFrwdBkwdPos]
  Md61PassStFwdBkwdTrgtPosCalib_TrgtPosArray_read/1 -> Demux1/1
  Demux1/2 -> Terminator2/1
  Demux1/1 -> [Md61PassStFwdBkwdTrgtPos]
  Demux1/3 -> Terminator3/1
  Demux3/1 -> [Md61ThdRwLtStFrwdBkwdPosTrgtPos]
  Demux3/3 -> Terminator7/1
  Demux3/2 -> Terminator6/1
  Md61ThdRwLtStFrwdBkwdPosTrgtPosCalib_TrgtPosArray_read/1 -> Demux3/1
  Demux4/1 -> [Md61ThdRwRtStFrwdBkwdPosTrgtPos]
  Demux4/3 -> Terminator9/1
  Demux4/2 -> Terminator8/1
  Md61ThdRwRtStFrwdBkwdPosTrgtPosCalib_TrgtPosArray_read/1 -> Demux4/1
  [ThdRwLtStFrwdBkwdPos] -> Relational Operator12/1
  [Md61ThdRwLtStFrwdBkwdPosTrgtPos] -> Add4/1
  Constant12/1 -> Add4/2
  Add4/1 -> Relational Operator12/2
  Logical Operator38/1 -> [Stage2Done], Md61Stage2DoneSecRwStReset_Val_write/1, Chart/23(Stage2Done)
  [Stage2Done] -> Unit Delay12/1, Logical Operator48/1
  Unit Delay12/1 -> Logical Operator49/1
  Logical Operator49/1 -> Logical Operator48/2
  Relational Operator12/1 -> Switch10/1
  [Stage2DoneTrig] -> Switch10/2
  Unit Delay13/1 -> Switch10/3
  Unit Delay14/1 -> Switch11/3
  [Stage2DoneTrig] -> Switch11/2
  Relational Operator13/1 -> Switch11/1
  Add5/1 -> Relational Operator13/2
  Constant13/1 -> Add5/2
  [Md61ThdRwRtStFrwdBkwdPosTrgtPos] -> Add5/1
  [ThdRwRtStFrwdBkwdPos] -> Relational Operator13/1
  [Md61PassStFwdBkwdTrgtPos] -> Add6/1
  PA_KeSMSuFirstRwStBackPosDelta_Val3/1 -> Add6/2
  Add6/1 -> Relational Operator14/2
  Relational Operator14/1 -> Switch12/1
  [Stage2DoneTrig] -> Switch12/2
  Unit Delay15/1 -> Switch12/3
  [IfVeSMSuPassStFrwdBkwdPos] -> Relational Operator14/1
  [PassStBkReclnPos] -> Relational Operator15/1
  Unit Delay16/1 -> Switch13/3
  [Stage2DoneTrig] -> Switch13/2
  Relational Operator15/1 -> Switch13/1
  Add8/1 -> Relational Operator15/2
  PA_KeSMSuFirstRwStBackPosDelta_Val2/1 -> Add8/2
  [Md61PassStBkReclnUpwdDnwdTrgtPos] -> Add8/1
  [Stage3ThdRwLtEn] -> Chart/24(Stage3ThdRwLtEn)
  [Stage3ThdRwRtEn] -> Chart/25(Stage3ThdRwRtEn)
  [Stage3PassStFwdBkwdEn] -> Chart/26(Stage3PassStFwdBkwdEn)
  [Stage3PassStBkEn] -> Chart/27(Stage3PassStBkEn)
  [Stage3ThdRwLtEn] -> Logical Operator50/1
  Logical Operator50/1 -> Logical Operator51/1
  [Stage3ThdRwRtEn] -> Logical Operator55/1
  [Stage3PassStFwdBkwdEn] -> Logical Operator56/1
  [Stage3PassStBkEn] -> Logical Operator57/1
  Logical Operator55/1 -> Logical Operator52/1
  Logical Operator56/1 -> Logical Operator53/1
  Logical Operator57/1 -> Logical Operator54/1
  [PassStBkReclnStgDone] -> Logical Operator54/2
  [PassStFwdBkwdStgDone] -> Logical Operator53/2
  [ThdRwRtStBkReclnStgDone] -> Logical Operator58/1
  [ThdRwRtStFwdBkwdStgDone] -> Logical Operator58/2
  Logical Operator58/1 -> Logical Operator52/2
  Logical Operator59/1 -> Logical Operator51/2
  [ThdRwLtStBkReclnStgDone] -> Logical Operator59/1
  [ThdRwLtStFwdBkwdStgDone] -> Logical Operator59/2
  Logical Operator51/1 -> Logical Operator60/1
  Logical Operator52/1 -> Logical Operator60/2
  Logical Operator53/1 -> Logical Operator60/3
  Logical Operator54/1 -> Logical Operator60/4
  Logical Operator60/1 -> [Stage3Done]
  [Stage3Done] -> Chart/28(Stage3Done)
  [SecRwLtStLgrstOtwdInwdStgDone] -> Logical Operator62/1
  [ZeroLStgDone] -> Logical Operator61/3
  [SecRwLtStFrwdBkwdStgDone] -> Logical Operator61/2
  [SecRwLtStBkReclnStgDone] -> Logical Operator61/1
  [SecRwLtStLgrstUpwdDnwdStgDone] -> Logical Operator62/2
  Logical Operator62/1 -> Logical Operator61/4
  Logical Operator61/1 -> [Stage4SecRwLtDone]
  [SecRwRtStFrwdBkwdStgDone] -> Logical Operator63/2
  Logical Operator64/1 -> Logical Operator63/3
  [ZeroRStgDone] -> Logical Operator63/4
  [SecRwRtStBkReclnStgDone] -> Logical Operator63/1
  [SecRwRtStLgrstUpwdDnwdStgDone] -> Logical Operator64/2
  [SecRwRtStLgrstOtwdInwdStgDone] -> Logical Operator64/1
  Logical Operator63/1 -> [Stage4SecRwRtDone]
  [Stage4SecRwLtDone] -> Logical Operator65/1
  [Stage4SecRwRtDone] -> Logical Operator65/2
  Logical Operator65/1 -> [Stage4Done]
  [Stage4Done] -> Chart/29(Stage4Done)
  [Stage2Done] -> Unit Delay19/1
  [Stage3Done] -> Logical Operator66/2
  [Stage4Done] -> Logical Operator66/3
  [PassStBkStgDone] -> Logical Operator66/4
  [PassStFwdBkwdStgDone] -> Logical Operator66/5
  [ThdRwLtStBkReclnStgDone] -> Logical Operator66/6
  [ThdRwLtStFwdBkwdStgDone] -> Logical Operator66/7
  [ThdRwRtStBkReclnStgDone] -> Logical Operator66/8
  [ThdRwRtStFwdBkwdStgDone] -> Logical Operator66/9
  Logical Operator66/1 -> [AllDone]
  IfVeSMSuSecRwLtStBkReclnUpwdDnwdPos_Val_read/1 -> [SecRwLtStBkReclnUpwdDnwdPos]
  IfVeSMSuSecRwLtStLgrstUpwdDnwdPos_Val_read/1 -> [SecRwLtStLgrstUpwdDnwdPos]
  IfVeSMSuSecRwLtStLgrstOtwdInwdPos_Val_read/1 -> [SecRwLtStLgrstOtwdInwdPos]
  IfVeSMSuSecRwLtStZeroPos_Val_read/1 -> [SecRwLtStZeroPos]
  IfVeSMSuSecRwRtStBkReclnUpwdDnwdPos_Val_read/1 -> [SecRwRtStBkReclnUpwdDnwdPos]
  IfVeSMSuSecRwRtStLgrstOtwdInwdPos_Val_read/1 -> [SecRwRtStLgrstOtwdInwdPos]
  IfVeSMSuSecRwRtStLgrstUpwdDnwdPos_Val_read/1 -> [SecRwRtStLgrstUpwdDnwdPos]
  IfVeSMSuSecRwRtStZeroPos_Val_read/1 -> [SecRwRtStZeroPos]
  Demux5/3 -> Terminator11/1
  Demux5/2 -> Terminator10/1
  Demux5/1 -> [Md61SecRwLtStBkReclnTrgtPos]
  Md61SecRwLtStBkReclnTrgtPosCalib_TrgtPosArray_read/1 -> Demux5/1
  Md61SecRwLtStCushFrntTrgtPosCalib_TrgtPosArray_read/1 -> Demux6/1
  Demux6/1 -> [Md61SecRwLtStCushFrntTrgtPos]
  Demux6/2 -> Terminator12/1
  Demux6/3 -> Terminator13/1
  Demux7/3 -> Terminator15/1
  Demux7/2 -> Terminator14/1
  Demux7/1 -> [Md61SecRwLtStLgrstInwdOtwdTrgtPos]
  Md61SecRwLtStLgrstInwdOtwdTrgtPosCalib_TrgtPosArray_read/1 -> Demux7/1
  Md61SecRwLtStLgrstUpwdDnwdTrgtPosCalib_TrgtPosArray_read/1 -> Demux8/1
  Demux8/1 -> [Md61SecRwLtStLgrstUpwdDnwdTrgtPos]
  Demux8/2 -> Terminator16/1
  Demux8/3 -> Terminator17/1
  Md61SecRwRtStBkReclnTrgtPosCalib_TrgtPosArray_read/1 -> Demux9/1
  Demux10/3 -> Terminator21/1
  Demux9/3 -> Terminator19/1
  Md61SecRwRtStCushFrntTrgtPosCalib_TrgtPosArray_read/1 -> Demux10/1
  Demux10/1 -> [Md61SecRwRtStCushFrntTrgtPos]
  Demux9/1 -> [Md61SecRwRtStBkReclnTrgtPos]
  Demux10/2 -> Terminator20/1
  Demux9/2 -> Terminator18/1
  Md61SecRwRtStLgrstInwdOtwdTrgtPosCalib_TrgtPosArray_read/1 -> Demux11/1
  Demux12/3 -> Terminator25/1
  Demux11/3 -> Terminator23/1
  Md61SecRwRtStLgrstUpwdDnwdTrgtPosCalib_TrgtPosArray_read/1 -> Demux12/1
  Demux12/1 -> [Md61SecRwRtStLgrstUpwdDnwdTrgtPos]
  Demux11/1 -> [Md61SecRwRtStLgrstInwdOtwdTrgtPos]
  Demux12/2 -> Terminator24/1
  Demux11/2 -> Terminator22/1
  [SecRwLtStBkReclnUpwdDnwdPos] -> Chart/30(IfVeSMSuSecRwLtStBkReclnUpwdDnwdPos)
  [SecRwLtStLgrstOtwdInwdPos] -> Chart/31(IfVeSMSuSecRwLtStLgrstOtwdInwdPos)
  [SecRwLtStLgrstUpwdDnwdPos] -> Chart/32(IfVeSMSuSecRwLtStLgrstUpwdDnwdPos)
  [SecRwLtStZeroPos] -> Chart/33(IfVeSMSuSecRwLtStZeroPos)
  [Md61SecRwLtStBkReclnTrgtPos] -> Chart/34(Ltbktrgt)
  [Md61SecRwLtStLgrstInwdOtwdTrgtPos] -> Chart/35(Ltlgrstintrgt)
  [Md61SecRwLtStCushFrntTrgtPos] -> Chart/37(Ltzerotrgt)
  [Md61SecRwLtStLgrstUpwdDnwdTrgtPos] -> Chart/36(Ltlgrstuptrgt)
  [SecRwLtStBkReclnStgDone] -> Chart/46(SecRwLtStBkReclnStgDone)
  [SecRwLtStFrwdBkwdStgDone] -> Chart/48(SecRwLtStFrwdBkwdStgDone)
  [SecRwLtStLgrstOtwdInwdStgDone] -> Chart/49(SecRwLtStLgrstOtwdInwdStgDone)
  [SecRwLtStLgrstUpwdDnwdStgDone] -> Chart/50(SecRwLtStLgrstUpwdDnwdStgDone)
  [ZeroLStgDone] -> Chart/47(ZeroLStgDone)
  [SecRwRtStBkReclnStgDone] -> Chart/51(SecRwRtStBkReclnStgDone)
  [ZeroRStgDone] -> Chart/52(ZeroRStgDone)
  [SecRwRtStLgrstUpwdDnwdStgDone] -> Chart/55(SecRwRtStLgrstUpwdDnwdStgDone)
  [SecRwRtStLgrstOtwdInwdStgDone] -> Chart/54(SecRwRtStLgrstOtwdInwdStgDone)
  [SecRwRtStFrwdBkwdStgDone] -> Chart/53(SecRwRtStFrwdBkwdStgDone)
  [SeatBkLimitPos] -> Chart/56(Md30PassStBkReclnTrgtPos1)
  Add2/1 -> [SeatBkLimitPosMinusDelt], Relational Operator6/2
  [SeatBkLimitPosMinusDelt] -> Relational Operator5/2
  [IfVeSMSuPassStFrwdBkwdPos] -> Chart/57(PassStFwdBkwdPos)
  [IfVeSMSuPassStFldUpwdDnwdPos] -> Chart/58(PassStFldUpwdDnwdPos)
  [Md61PassStBkReclnUpwdDnwdTrgtPos] -> Chart/59(Md61PassStBkReclnTrgtPos)
  [Stage2Done] -> Logical Operator67/2
  [FirstTrig] -> Logical Operator67/1
  Logical Operator48/1 -> Logical Operator68/1
  Logical Operator67/1 -> Logical Operator68/2
  Logical Operator68/1 -> [Stage2DoneTrig]
  Switch14/1 -> Unit Delay13/1, [Stage3ThdRwLtEn]
  Switch10/1 -> Switch14/3
  [FirstTrig] -> Logical Operator69/1
  [Stage2Done] -> Logical Operator70/1
  Logical Operator70/1 -> Logical Operator69/2
  Logical Operator69/1 -> Switch17/2, Switch16/2, Switch15/2, Switch14/2
  Constant16/1 -> Switch14/1
  Switch11/1 -> Switch15/3
  Switch15/1 -> [Stage3ThdRwRtEn], Unit Delay14/1
  Constant17/1 -> Switch15/1
  Switch12/1 -> Switch16/3
  Constant18/1 -> Switch16/1
  Switch16/1 -> Unit Delay15/1, [Stage3PassStFwdBkwdEn]
  Switch13/1 -> Switch17/3
  Switch17/1 -> Unit Delay16/1, [Stage3PassStBkEn]
  Constant19/1 -> Switch17/1
  Switch18/1 -> Switch3/1
  Constant20/1 -> Switch18/3
  Switch19/1 -> Switch2/1
  Relational Operator/1 -> Switch19/1, Switch19/2
  Constant22/1 -> Switch19/3
  Switch20/1 -> Switch4/1
  Relational Operator2/1 -> Switch20/1, Switch20/2
  Constant23/1 -> Switch20/3
  Switch21/1 -> Switch5/1
  Relational Operator3/1 -> Switch21/1, Switch21/2
  Constant24/1 -> Switch21/3
  Switch22/1 -> Switch6/1
  Logical Operator31/1 -> Switch22/1, Switch22/2
  Constant25/1 -> Switch22/3
  Switch23/1 -> Switch7/1
  Constant26/1 -> Switch23/3
  [SecRwRtStBkReclnUpwdDnwdPos] -> Chart/38(IfVeSMSuSecRwRtStBkReclnUpwdDnwdPos)
  [SecRwRtStLgrstOtwdInwdPos] -> Chart/39(IfVeSMSuSecRwRtStLgrstOtwdInwdPos)
  [SecRwRtStLgrstUpwdDnwdPos] -> Chart/40(IfVeSMSuSecRwRtStLgrstUpwdDnwdPos)
  [SecRwRtStZeroPos] -> Chart/41(IfVeSMSuSecRwRtStZeroPos)
  [Md61SecRwRtStBkReclnTrgtPos] -> Chart/42(Rtbktrgt)
  [Md61SecRwRtStLgrstInwdOtwdTrgtPos] -> Chart/43(Rtlgrstintrgt)
  [Md61SecRwRtStLgrstUpwdDnwdTrgtPos] -> Chart/44(Rtlgrstuptrgt)
  [Md61SecRwRtStCushFrntTrgtPos] -> Chart/45(Rtzerotrgt)
  Unit Delay19/1 -> Logical Operator66/1
  [FirstTrig] -> Logical Operator71/1
  Logical Operator71/1 -> Logical Operator66/10
  Relational Operator4/1 -> Logical Operator32/1
  Logical Operator32/1 -> Switch23/1, Switch23/2
  [FirstTrig] -> Logical Operator72/1
  Logical Operator72/1 -> Logical Operator73/2
  Logical Operator36/1 -> Logical Operator73/1
  Logical Operator33/1 -> Logical Operator74/1
  Logical Operator37/1 -> Logical Operator36/1
  Unit Delay17/1 -> Logical Operator36/2
  Unit Delay18/1 -> Logical Operator36/3
  Logical Operator73/1 -> Logical Operator74/2
  Logical Operator74/1 -> [Stage2PassStDone]
  PA_KeSMSuThrdRwCushFoldPosDelta_Val/1 -> Relational Operator/2
  PA_KeSMSuThrdRwCushFoldPosDelta_Val2/1 -> Divide/1
  Constant4/1 -> Divide/2
  Divide/1 -> Relational Operator2/2
  Constant5/1 -> Divide1/2
  PA_KeSMSuThrdRwCushFoldPosDelta_Val3/1 -> Divide1/1

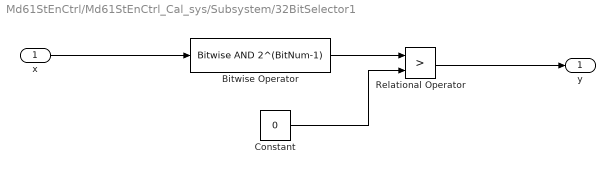
== system Md61StEnCtrl/Md61StEnCtrl_Cal_sys/Subsystem/32BitSelector1 ==
  x : Inport
  Bitwise Operator : simulink/Logic and Bit Operations/Bitwise Operator  logicop=AND  UseBitMask=on  BitMask=2^(BitNum-1)  BitMaskRealWorld=Stored Integer
  Constant : Constant  Value=0  OutDataTypeStr=uint32
  Relational Operator : RelationalOperator  Operator=>  OutDataTypeStr=boolean  RndMeth=Simplest
  y : Outport
  wires:
  Relational Operator/1 -> y/1
  Constant/1 -> Relational Operator/2
  x/1 -> Bitwise Operator/1
  Bitwise Operator/1 -> Relational Operator/1

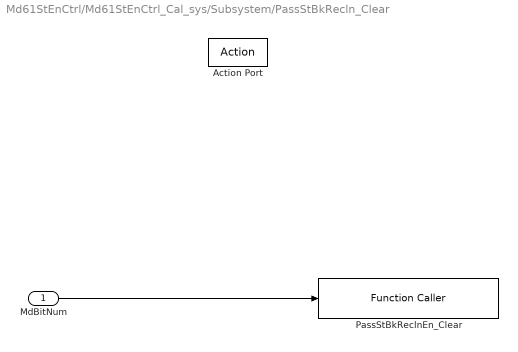
== system Md61StEnCtrl/Md61StEnCtrl_Cal_sys/Subsystem/PassStBkRecln_Clear ==
  MdBitNum : Inport
  Action Port : ActionPort  ActionType=else
  PassStBkReclnEn_Clear : FunctionCaller  FunctionPrototype=PassStBkReclnEn_Clear(data)  InputArgumentSpecifications=uint8(1)
  wires:
  MdBitNum/1 -> PassStBkReclnEn_Clear/1

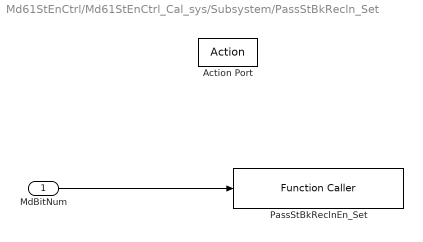
== system Md61StEnCtrl/Md61StEnCtrl_Cal_sys/Subsystem/PassStBkRecln_Set ==
  MdBitNum : Inport
  Action Port : ActionPort  ActionType=then
  PassStBkReclnEn_Set : FunctionCaller  FunctionPrototype=PassStBkReclnEn_Set(data)  InputArgumentSpecifications=uint8(1)
  wires:
  MdBitNum/1 -> PassStBkReclnEn_Set/1

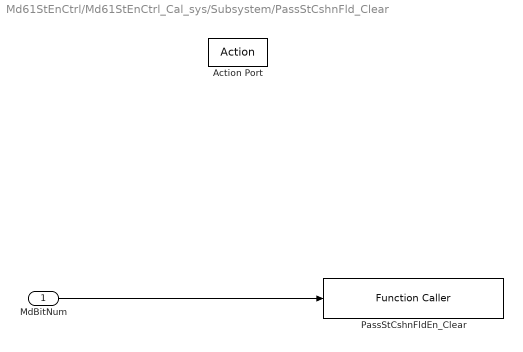
== system Md61StEnCtrl/Md61StEnCtrl_Cal_sys/Subsystem/PassStCshnFld_Clear ==
  MdBitNum : Inport
  Action Port : ActionPort  ActionType=else
  PassStCshnFldEn_Clear : FunctionCaller  FunctionPrototype=PassStCshnFldEn_Clear(data)  InputArgumentSpecifications=uint8(1)
  wires:
  MdBitNum/1 -> PassStCshnFldEn_Clear/1

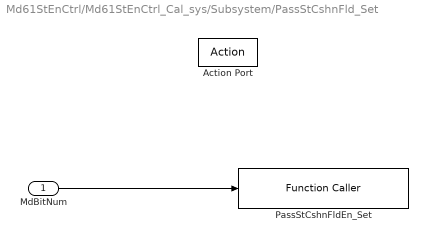
== system Md61StEnCtrl/Md61StEnCtrl_Cal_sys/Subsystem/PassStCshnFld_Set ==
  MdBitNum : Inport
  Action Port : ActionPort  ActionType=then
  PassStCshnFldEn_Set : FunctionCaller  FunctionPrototype=PassStCshnFldEn_Set(data)  InputArgumentSpecifications=uint8(1)
  wires:
  MdBitNum/1 -> PassStCshnFldEn_Set/1

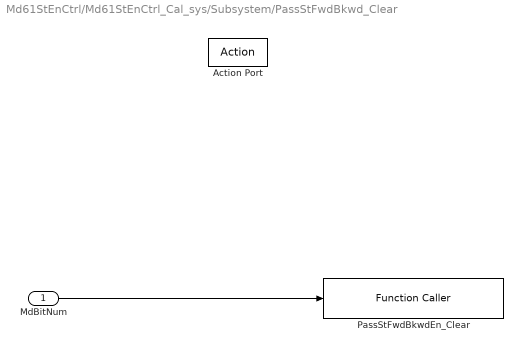
== system Md61StEnCtrl/Md61StEnCtrl_Cal_sys/Subsystem/PassStFwdBkwd_Clear ==
  MdBitNum : Inport
  Action Port : ActionPort  ActionType=else
  PassStFwdBkwdEn_Clear : FunctionCaller  FunctionPrototype=PassStFwdBkwdEn_Clear(data)  InputArgumentSpecifications=uint8(1)
  wires:
  MdBitNum/1 -> PassStFwdBkwdEn_Clear/1

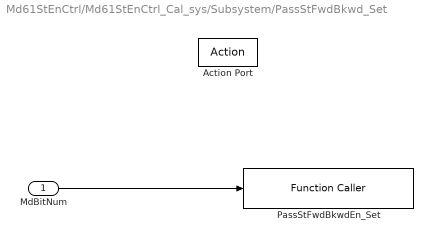
== system Md61StEnCtrl/Md61StEnCtrl_Cal_sys/Subsystem/PassStFwdBkwd_Set ==
  MdBitNum : Inport
  Action Port : ActionPort  ActionType=then
  PassStFwdBkwdEn_Set : FunctionCaller  FunctionPrototype=PassStFwdBkwdEn_Set(data)  InputArgumentSpecifications=uint8(1)
  wires:
  MdBitNum/1 -> PassStFwdBkwdEn_Set/1

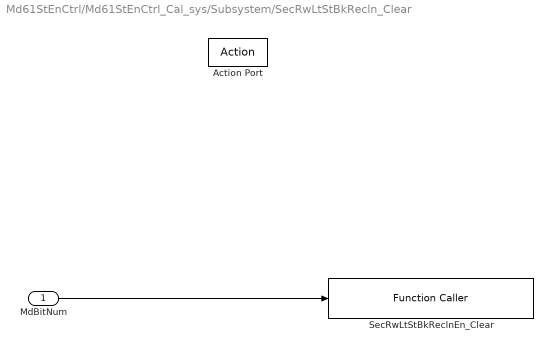
== system Md61StEnCtrl/Md61StEnCtrl_Cal_sys/Subsystem/SecRwLtStBkRecln_Clear ==
  MdBitNum : Inport
  Action Port : ActionPort  ActionType=else
  SecRwLtStBkReclnEn_Clear : FunctionCaller  FunctionPrototype=SecRwLtStBkReclnEn_Clear(data)  InputArgumentSpecifications=uint8(1)
  wires:
  MdBitNum/1 -> SecRwLtStBkReclnEn_Clear/1

== system Md61StEnCtrl/Md61StEnCtrl_Cal_sys/Subsystem/SecRwLtStBkRecln_Set ==
  MdBitNum : Inport
  Action Port : ActionPort  ActionType=then
  SecRwLtStBkReclnEn_Set : FunctionCaller  FunctionPrototype=SecRwLtStBkReclnEn_Set(data)  InputArgumentSpecifications=uint8(1)
  wires:
  MdBitNum/1 -> SecRwLtStBkReclnEn_Set/1

== system Md61StEnCtrl/Md61StEnCtrl_Cal_sys/Subsystem/SecRwLtStFwdBkwd_Clear ==
  MdBitNum : Inport
  Action Port : ActionPort  ActionType=else
  SecRwLtStFwdBkwdEn_Clear : FunctionCaller  FunctionPrototype=SecRwLtStFwdBkwdEn_Clear(data)  InputArgumentSpecifications=uint8(1)
  wires:
  MdBitNum/1 -> SecRwLtStFwdBkwdEn_Clear/1

== system Md61StEnCtrl/Md61StEnCtrl_Cal_sys/Subsystem/SecRwLtStFwdBkwd_Set ==
  MdBitNum : Inport
  Action Port : ActionPort  ActionType=then
  SecRwLtStFwdBkwdEn_Set : FunctionCaller  FunctionPrototype=SecRwLtStFwdBkwdEn_Set(data)  InputArgumentSpecifications=uint8(1)
  wires:
  MdBitNum/1 -> SecRwLtStFwdBkwdEn_Set/1

== system Md61StEnCtrl/Md61StEnCtrl_Cal_sys/Subsystem/SecRwLtStLgrstInwdOtwd_Clear ==
  MdBitNum : Inport
  Action Port : ActionPort  ActionType=else
  SecRwLtStLgrstInwdOtwdEn_Clear : FunctionCaller  FunctionPrototype=SecRwLtStLgrstInwdOtwdEn_Clear(data)  InputArgumentSpecifications=uint8(1)
  wires:
  MdBitNum/1 -> SecRwLtStLgrstInwdOtwdEn_Clear/1

== system Md61StEnCtrl/Md61StEnCtrl_Cal_sys/Subsystem/SecRwLtStLgrstInwdOtwd_Set ==
  MdBitNum : Inport
  Action Port : ActionPort  ActionType=then
  SecRwLtStLgrstInwdOtwdEn_Set : FunctionCaller  FunctionPrototype=SecRwLtStLgrstInwdOtwdEn_Set(data)  InputArgumentSpecifications=uint8(1)
  wires:
  MdBitNum/1 -> SecRwLtStLgrstInwdOtwdEn_Set/1

== system Md61StEnCtrl/Md61StEnCtrl_Cal_sys/Subsystem/SecRwLtStLgrstUpwdDnwd_Clear ==
  MdBitNum : Inport
  Action Port : ActionPort  ActionType=else
  SecRwLtStLgrstUpwdDnwdEn_Clear : FunctionCaller  FunctionPrototype=SecRwLtStLgrstUpwdDnwdEn_Clear(data)  InputArgumentSpecifications=uint8(1)
  wires:
  MdBitNum/1 -> SecRwLtStLgrstUpwdDnwdEn_Clear/1

== system Md61StEnCtrl/Md61StEnCtrl_Cal_sys/Subsystem/SecRwLtStLgrstUpwdDnwd_Set ==
  MdBitNum : Inport
  Action Port : ActionPort  ActionType=then
  SecRwLtStLgrstUpwdDnwdEn_Set : FunctionCaller  FunctionPrototype=SecRwLtStLgrstUpwdDnwdEn_Set(data)  InputArgumentSpecifications=uint8(1)
  wires:
  MdBitNum/1 -> SecRwLtStLgrstUpwdDnwdEn_Set/1

== system Md61StEnCtrl/Md61StEnCtrl_Cal_sys/Subsystem/SecRwRtStBkRecln_Clear ==
  MdBitNum : Inport
  Action Port : ActionPort  ActionType=else
  SecRwRtStBkReclnEn_Clear : FunctionCaller  FunctionPrototype=SecRwRtStBkReclnEn_Clear(data)  InputArgumentSpecifications=uint8(1)
  wires:
  MdBitNum/1 -> SecRwRtStBkReclnEn_Clear/1

== system Md61StEnCtrl/Md61StEnCtrl_Cal_sys/Subsystem/SecRwRtStBkRecln_Set ==
  MdBitNum : Inport
  Action Port : ActionPort  ActionType=then
  SecRwRtStBkReclnEn_Set : FunctionCaller  FunctionPrototype=SecRwRtStBkReclnEn_Set(data)  InputArgumentSpecifications=uint8(1)
  wires:
  MdBitNum/1 -> SecRwRtStBkReclnEn_Set/1

== system Md61StEnCtrl/Md61StEnCtrl_Cal_sys/Subsystem/SecRwRtStFwdBkwd_Clear ==
  MdBitNum : Inport
  Action Port : ActionPort  ActionType=else
  SecRwRtStFwdBkwdEn_Clear : FunctionCaller  FunctionPrototype=SecRwRtStFwdBkwdEn_Clear(data)  InputArgumentSpecifications=uint8(1)
  wires:
  MdBitNum/1 -> SecRwRtStFwdBkwdEn_Clear/1

== system Md61StEnCtrl/Md61StEnCtrl_Cal_sys/Subsystem/SecRwRtStFwdBkwd_Set ==
  MdBitNum : Inport
  Action Port : ActionPort  ActionType=then
  SecRwRtStFwdBkwdEn_Set : FunctionCaller  FunctionPrototype=SecRwRtStFwdBkwdEn_Set(data)  InputArgumentSpecifications=uint8(1)
  wires:
  MdBitNum/1 -> SecRwRtStFwdBkwdEn_Set/1

== system Md61StEnCtrl/Md61StEnCtrl_Cal_sys/Subsystem/SecRwRtStLgrstInwdOtwd_Clear ==
  MdBitNum : Inport
  Action Port : ActionPort  ActionType=else
  SecRwRtStLgrstInwdOtwdEn_Clear : FunctionCaller  FunctionPrototype=SecRwRtStLgrstInwdOtwdEn_Clear(data)  InputArgumentSpecifications=uint8(1)
  wires:
  MdBitNum/1 -> SecRwRtStLgrstInwdOtwdEn_Clear/1

== system Md61StEnCtrl/Md61StEnCtrl_Cal_sys/Subsystem/SecRwRtStLgrstInwdOtwd_Set ==
  MdBitNum : Inport
  Action Port : ActionPort  ActionType=then
  SecRwRtStLgrstInwdOtwdEn_Set : FunctionCaller  FunctionPrototype=SecRwRtStLgrstInwdOtwdEn_Set(data)  InputArgumentSpecifications=uint8(1)
  wires:
  MdBitNum/1 -> SecRwRtStLgrstInwdOtwdEn_Set/1

== system Md61StEnCtrl/Md61StEnCtrl_Cal_sys/Subsystem/SecRwRtStLgrstUpwdDnwd_Clear ==
  MdBitNum : Inport
  Action Port : ActionPort  ActionType=else
  SecRwRtStLgrstUpwdDnwdEn_Clear : FunctionCaller  FunctionPrototype=SecRwRtStLgrstUpwdDnwdEn_Clear(data)  InputArgumentSpecifications=uint8(1)
  wires:
  MdBitNum/1 -> SecRwRtStLgrstUpwdDnwdEn_Clear/1

== system Md61StEnCtrl/Md61StEnCtrl_Cal_sys/Subsystem/SecRwRtStLgrstUpwdDnwd_Set ==
  MdBitNum : Inport
  Action Port : ActionPort  ActionType=then
  SecRwRtStLgrstUpwdDnwdEn_Set : FunctionCaller  FunctionPrototype=SecRwRtStLgrstUpwdDnwdEn_Set(data)  InputArgumentSpecifications=uint8(1)
  wires:
  MdBitNum/1 -> SecRwRtStLgrstUpwdDnwdEn_Set/1

== system Md61StEnCtrl/Md61StEnCtrl_Cal_sys/Subsystem/ThdRwLtStBkRecln_Clear ==
  MdBitNum : Inport
  Action Port : ActionPort  ActionType=else
  ThdRwLtStBkReclnEn_Clear : FunctionCaller  FunctionPrototype=ThdRwLtStBkReclnEn_Clear(data)  InputArgumentSpecifications=uint8(1)
  wires:
  MdBitNum/1 -> ThdRwLtStBkReclnEn_Clear/1

== system Md61StEnCtrl/Md61StEnCtrl_Cal_sys/Subsystem/ThdRwLtStBkRecln_Set ==
  MdBitNum : Inport
  Action Port : ActionPort  ActionType=then
  ThdRwLtStBkReclnEn_Set : FunctionCaller  FunctionPrototype=ThdRwLtStBkReclnEn_Set(data)  InputArgumentSpecifications=uint8(1)
  wires:
  MdBitNum/1 -> ThdRwLtStBkReclnEn_Set/1

== system Md61StEnCtrl/Md61StEnCtrl_Cal_sys/Subsystem/ThdRwLtStCshnFld_Clear ==
  MdBitNum : Inport
  Action Port : ActionPort  ActionType=else
  ThdRwLtStCshnFldEn_Clear : FunctionCaller  FunctionPrototype=ThdRwLtStCshnFldEn_Clear(data)  InputArgumentSpecifications=uint8(1)
  wires:
  MdBitNum/1 -> ThdRwLtStCshnFldEn_Clear/1

== system Md61StEnCtrl/Md61StEnCtrl_Cal_sys/Subsystem/ThdRwLtStCshnFld_Set ==
  MdBitNum : Inport
  Action Port : ActionPort  ActionType=then
  ThdRwLtStCshnFldEn_Set : FunctionCaller  FunctionPrototype=ThdRwLtStCshnFldEn_Set(data)  InputArgumentSpecifications=uint8(1)
  wires:
  MdBitNum/1 -> ThdRwLtStCshnFldEn_Set/1

== system Md61StEnCtrl/Md61StEnCtrl_Cal_sys/Subsystem/ThdRwLtStFwdBkwd_Clear ==
  MdBitNum : Inport
  Action Port : ActionPort  ActionType=else
  ThdRwLtStFwdBkwdEn_Clear : FunctionCaller  FunctionPrototype=ThdRwLtStFwdBkwdEn_Clear(data)  InputArgumentSpecifications=uint8(1)
  wires:
  MdBitNum/1 -> ThdRwLtStFwdBkwdEn_Clear/1

== system Md61StEnCtrl/Md61StEnCtrl_Cal_sys/Subsystem/ThdRwLtStFwdBkwd_Set ==
  MdBitNum : Inport
  Action Port : ActionPort  ActionType=then
  ThdRwLtStFwdBkwdEn_Set : FunctionCaller  FunctionPrototype=ThdRwLtStFwdBkwdEn_Set(data)  InputArgumentSpecifications=uint8(1)
  wires:
  MdBitNum/1 -> ThdRwLtStFwdBkwdEn_Set/1

== system Md61StEnCtrl/Md61StEnCtrl_Cal_sys/Subsystem/ThdRwRtStBkRecln_Clear ==
  MdBitNum : Inport
  Action Port : ActionPort  ActionType=else
  ThdRwRtStBkReclnEn_Clear : FunctionCaller  FunctionPrototype=ThdRwRtStBkReclnEn_Clear(data)  InputArgumentSpecifications=uint8(1)
  wires:
  MdBitNum/1 -> ThdRwRtStBkReclnEn_Clear/1

== system Md61StEnCtrl/Md61StEnCtrl_Cal_sys/Subsystem/ThdRwRtStBkRecln_Set ==
  MdBitNum : Inport
  Action Port : ActionPort  ActionType=then
  ThdRwRtStBkReclnEn_Set : FunctionCaller  FunctionPrototype=ThdRwRtStBkReclnEn_Set(data)  InputArgumentSpecifications=uint8(1)
  wires:
  MdBitNum/1 -> ThdRwRtStBkReclnEn_Set/1

== system Md61StEnCtrl/Md61StEnCtrl_Cal_sys/Subsystem/ThdRwRtStCshnFld_Clear ==
  MdBitNum : Inport
  Action Port : ActionPort  ActionType=else
  ThdRwRtStCshnFldEn_Clear : FunctionCaller  FunctionPrototype=ThdRwRtStCshnFldEn_Clear(data)  InputArgumentSpecifications=uint8(1)
  wires:
  MdBitNum/1 -> ThdRwRtStCshnFldEn_Clear/1

== system Md61StEnCtrl/Md61StEnCtrl_Cal_sys/Subsystem/ThdRwRtStCshnFld_Set ==
  MdBitNum : Inport
  Action Port : ActionPort  ActionType=then
  ThdRwRtStCshnFldEn_Set : FunctionCaller  FunctionPrototype=ThdRwRtStCshnFldEn_Set(data)  InputArgumentSpecifications=uint8(1)
  wires:
  MdBitNum/1 -> ThdRwRtStCshnFldEn_Set/1

== system Md61StEnCtrl/Md61StEnCtrl_Cal_sys/Subsystem/ThdRwRtStFwdBkwd_Clear ==
  MdBitNum : Inport
  Action Port : ActionPort  ActionType=else
  ThdRwRtStFwdBkwdEn_Clear : FunctionCaller  FunctionPrototype=ThdRwRtStFwdBkwdEn_Clear(data)  InputArgumentSpecifications=uint8(1)
  wires:
  MdBitNum/1 -> ThdRwRtStFwdBkwdEn_Clear/1

== system Md61StEnCtrl/Md61StEnCtrl_Cal_sys/Subsystem/ThdRwRtStFwdBkwd_Set ==
  MdBitNum : Inport
  Action Port : ActionPort  ActionType=then
  ThdRwRtStFwdBkwdEn_Set : FunctionCaller  FunctionPrototype=ThdRwRtStFwdBkwdEn_Set(data)  InputArgumentSpecifications=uint8(1)
  wires:
  MdBitNum/1 -> ThdRwRtStFwdBkwdEn_Set/1
